simulink model "discretefilter_test_template"  (Simulink 8.4)
settings: Solver=VariableStepDiscrete  StartTime=0.0  StopTime=10.0  MaxStep=1  RelTol=1e-3
settings Model: Creator=arnaud  LastModifiedBy=arnaud
settings DataIOCC: ExternalInput=xin  SaveFormat=StructureWithTime

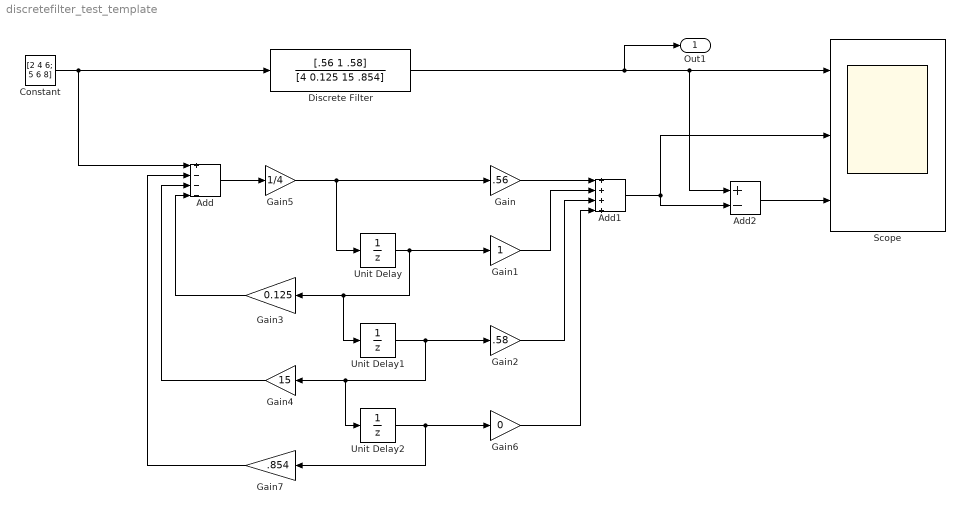
== system discretefilter_test_template ==
  Add : Sum  Inputs=+---
  Add1 : Sum  Inputs=++++
  Add2 : Sum  Inputs=+-
  Constant : Constant  Value=[2 4 6; 5 6 8]
  Discrete Filter : DiscreteFilter  Numerator=[.56 1 .58]  Denominator=[4 0.125 15 .854]  InitialStates=[0 1 5]  SampleTime=1
  Gain : Gain  Gain=.56
  Gain1 : Gain
  Gain2 : Gain  Gain=.58
  Gain3 : Gain  Gain=0.125
  Gain4 : Gain  Gain=15
  Gain5 : Gain  Gain=1/4
  Gain6 : Gain  Gain=0
  Gain7 : Gain  Gain=.854
  Scope : Scope  NumInputPorts=3
      settings: YMin=-5~-5~-5  YMax=5~5~5
  Unit Delay : UnitDelay  SampleTime=-1
  Unit Delay1 : UnitDelay  InitialCondition=1  SampleTime=-1
  Unit Delay2 : UnitDelay  InitialCondition=5  SampleTime=-1
  Out1 : Outport
  wires:
  Discrete Filter/1 -> Out1/1, Scope/1, Add2/1
  Unit Delay/1 -> Gain1/1, Unit Delay1/1, Gain3/1
  Add1/1 -> Scope/2, Add2/2
  Add2/1 -> Scope/3
  Gain/1 -> Add1/1
  Gain1/1 -> Add1/2
  Gain2/1 -> Add1/3
  Unit Delay1/1 -> Unit Delay2/1, Gain4/1, Gain2/1
  Gain3/1 -> Add/4
  Gain4/1 -> Add/3
  Add/1 -> Gain5/1
  Constant/1 -> Add/1, Discrete Filter/1
  Gain5/1 -> Gain/1, Unit Delay/1
  Unit Delay2/1 -> Gain7/1, Gain6/1
  Gain6/1 -> Add1/4
  Gain7/1 -> Add/2
